simulink model "msd_05_Simscape_1"  (R2014a)
settings: Solver=ode45  StartTime=0.0  StopTime=10.0  MaxStep=0.01  RelTol=1e-3
InitFcn:
  | m = 3.600;     % kg
  | k = 400;    % N/m
  | b = 10;      % Ns/m
libraries: fl_lib x4
Description:
  | Copyright 2014 The MathWorks, Inc.
settings Model: Creator=smiller  LastModifiedBy=smiller
settings DebuggingCC: UnderspecifiedInitializationDetection=Classic  StateNameClashWarn=warning

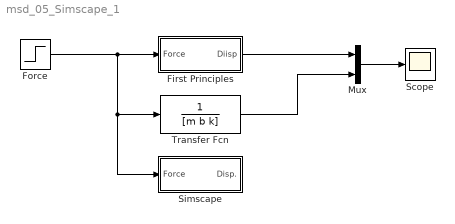
== system msd_05_Simscape_1 ==
  First Principles : Subsystem
  Force : Step  After=10  SampleTime=0
  Mux : Mux  Inputs=2
  Scope : Scope
  Simscape : Subsystem
  Transfer Fcn : TransferFcn  Denominator=[m b k]
  wires:
  Force/1 -> Simscape/1(Force), Transfer Fcn/1, First Principles/1(Force)
  First Principles/1(Diisp) -> Mux/1
  Mux/1 -> Scope/1
  Transfer Fcn/1 -> Mux/2

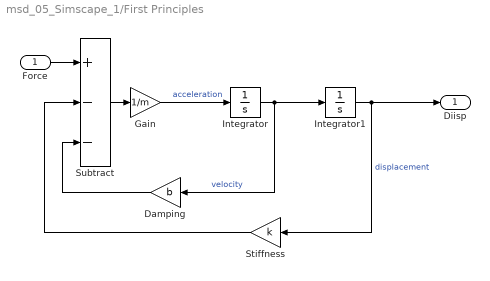
== system msd_05_Simscape_1/First Principles ==
  Force : Inport
  Damping : Gain  Gain=b
  Gain : Gain  Gain=1/m
  Integrator : Integrator
  Integrator1 : Integrator
  Stiffness : Gain  Gain=k
  Subtract : Sum  Inputs=+--
  Diisp : Outport
  wires:
  Force/1 -> Subtract/1
  Subtract/1 -> Gain/1
  Integrator/1 -> Damping/1, Integrator1/1  "velocity"
  Stiffness/1 -> Subtract/2
  Integrator1/1 -> Diisp/1, Stiffness/1  "displacement"
  Gain/1 -> Integrator/1  "acceleration"
  Damping/1 -> Subtract/3

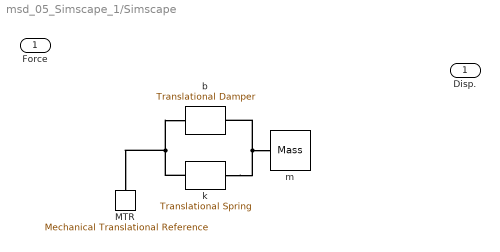
== system msd_05_Simscape_1/Simscape ==
  Force : Inport
  MTR : fl_lib/Mechanical/Translational Elements/Mechanical Translational Reference  f_Log=off  LocalVarNames=|f  LocalVarDescs=|f  LocalVarLogging=[]
  b : fl_lib/Mechanical/Translational Elements/Translational Damper  D=b N/(m/s)  f_Log=off  v_Log=off  LocalVarNames=|force|rel_velocity|power  LocalVarDescs=|Damping force (N)|Damper relative velocity (m/s)|Power dissipated in the damper (W)  LocalVarLogging=[0 0 0]
  k : fl_lib/Mechanical/Translational Elements/Translational Spring  spr_rate=k N/m  init_def=0 m  f_Log=off  v_Log=off  x_Log=off  LocalVarNames=|force|deformation  LocalVarDescs=|Spring force (N)|Spring deformation (m)  LocalVarLogging=[0 0]
  m : fl_lib/Mechanical/Translational Elements/Mass  mass=m kg  initial_velocity=0 m/s  f_Log=off  LocalVarNames=|force|velocity  LocalVarDescs=|Inertia force (N)|Mass absolute velocity (m/s)  LocalVarLogging=[0 0]
  Disp. : Outport
  connections:
  k/LConn1 -- b/LConn1 -- MTR/LConn1
  k/RConn1 -- m/LConn1 -- b/RConn1
